simulink model "FinalDemo2021b"  (R2023a)
settings: Solver=VariableStepAuto  StartTime=0.0  StopTime=inf  RelTol=1e-3
settings Model: Creator=bryantboatright  LastModifiedBy=boater

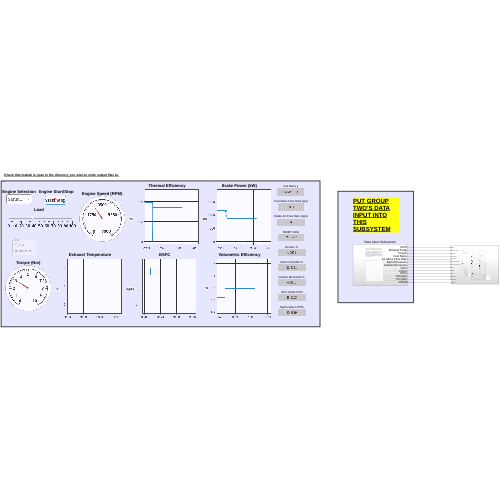
[thumbnail: Simulink's stored preview of the top-level diagram]
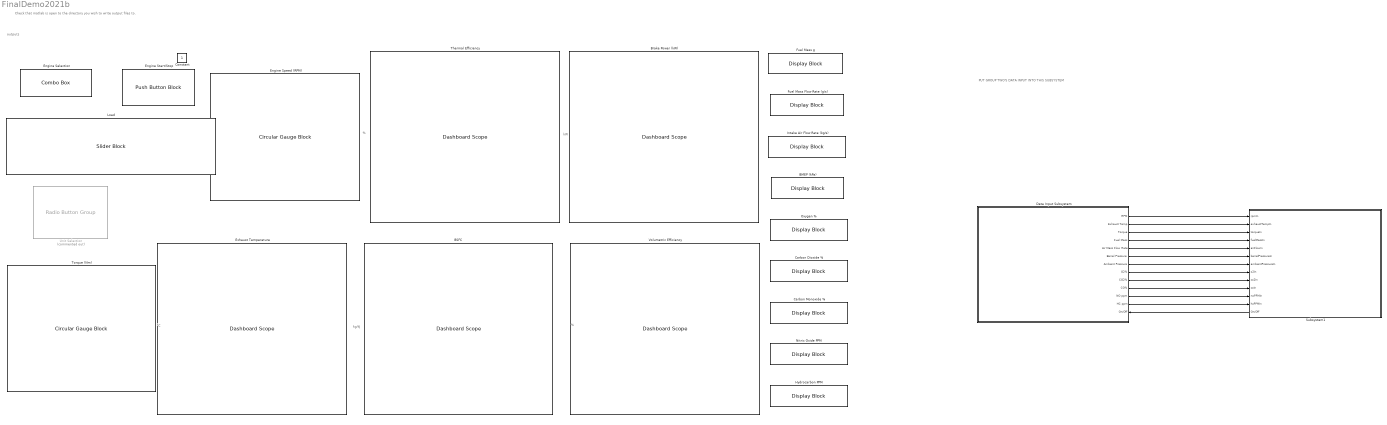
== system FinalDemo2021b ==
  note: %
  note: Check that matlab is open to the directory you wish to write output files to.
  note: PUT GROUP TWO'S DATA INPUT INTO THIS SUBSYSTEM
  note: ˚C
  note: kg/kJ
  note: kW
  note: outputs
  note: %
  BMEP (kPa) : DisplayBlock  LabelPosition=Hide  Transparency=1
  BSFC : DashboardScope  LegendPosition=Hide  UpdateMode=Scroll
  Brake Power (kW) : DashboardScope  LegendPosition=Hide  UpdateMode=Scroll
  Carbon Dioxide % : DisplayBlock  LabelPosition=Hide  Transparency=1
  Carbon Monoxide % : DisplayBlock  LabelPosition=Hide  Transparency=1
  Data Input Subsystem : Subsystem
      settings: PortSchema="{\"entries\":[{\"content\":{\"sides\":[{\"content\":{\"connectorIds\":[]},\"type\":\"ConnectorPlacement.EquallySpacedRectSide\",\"uuid\":\"3754a3e3-4518-42e3-a0cd-0eb816f7e60c\"},{\"content\":{\"connectorIds\":[\"Out1\",\"Out2\",\"Out3\",\"Out4\",\"Out5\",\"Out6\",\"Out7\",\"Out8\",\"Out9\",\"Out10\",\"Out11\",\"Out12\",\"In1\"],\"side\":\"RIGHT\"},\"type\":\"ConnectorPlacement.EquallySpacedRectSide\",\"uuid\":\"d3dfe676-b6e6-4c7f-98c7-8b108f201c07\"},{\"content\":{\"connectorIds\":[],\"side\":\"TOP\"},\"type\":\"ConnectorPlacement.EquallySpacedRectSide\",\"uuid\":\"2f91c8dd-0198-445b-930d-495fc8bcc849\"}]},\"type\":\"ConnectorPlacement.EquallySpacedConnector\",\"uuid\":\"520c6fba-fa44-47d2-96c9-29e04e3d0d93\"}],\"packageUris\":[\"http://schema.mathworks.com/mf0/Connector/R2020b\"],\"version\":\"1.0\"}"
  Engine Selection : ComboBox  LabelPosition=Hide  SelectedLabel=Yanmar
      settings: Values={{'Yanmar', 'Craftsman', 'John Deer', 'Chevy V6', 'Kohler', 'DuroMax'}, [1 2 3 4 5 6]}
  Engine Speed (RPM) : CircularGaugeBlock  LabelPosition=Hide  ScaleMax=7000  TickInterval=1750
  Engine Start/Stop : PushButtonBlock  ButtonText=Start/Stop  ButtonType=Latch  Icon=Engine  IconAlignment=Center  IconColor=On  OffValue=0.000000
  Exhaust Temperature : DashboardScope  LegendPosition=Hide  ScaleAtStop=off
  Fuel Mass Flow Rate (g/s) : DisplayBlock  LabelPosition=Hide  Transparency=1
  Fuel Mass g : DisplayBlock  LabelPosition=Hide  Transparency=1
  Hydrocarbon PPM : DisplayBlock  LabelPosition=Hide  Transparency=1
  Intake Air Flow Rate (kg/s) : DisplayBlock  LabelPosition=Hide  Transparency=1
  Load : SliderBlock  LabelPosition=Hide
  Nitric Oxide PPM : DisplayBlock  LabelPosition=Hide  Transparency=1
  Oxygen % : DisplayBlock  LabelPosition=Hide  Transparency=1
  Subsystem1 : Subsystem
      settings: PortSchema="{\"entries\":[{\"content\":{\"sides\":[{\"content\":{\"connectorIds\":[\"In1\",\"In2\",\"In3\",\"In4\",\"In5\",\"In6\",\"In7\",\"In8\",\"In9\",\"In10\",\"In11\",\"In12\",\"Out1\"]},\"type\":\"ConnectorPlacement.EquallySpacedRectSide\",\"uuid\":\"2e8fbbbd-04f3-4cfb-b1cc-1db1e48dc879\"},{\"content\":{\"connectorIds\":[],\"side\":\"RIGHT\"},\"type\":\"ConnectorPlacement.EquallySpacedRectSide\",\"uuid\":\"1e86395c-1e99-406b-884b-92366c924b1f\"},{\"content\":{\"connectorIds\":[],\"side\":\"TOP\"},\"type\":\"ConnectorPlacement.EquallySpacedRectSide\",\"uuid\":\"23f1f2f5-9354-4dfe-ba19-9e9e16993f9b\"}]},\"type\":\"ConnectorPlacement.EquallySpacedConnector\",\"uuid\":\"bb08251b-5f96-4a99-a638-0e0833315a09\"}],\"packageUris\":[\"http://schema.mathworks.com/mf0/Connector/R2020b\"],\"version\":\"1.0\"}"
  Thermal Efficiency : DashboardScope  LegendPosition=Hide  UpdateMode=Scroll
  Torque (Nm) : CircularGaugeBlock  LabelPosition=Hide  ScaleMax=10  TickInterval=1
  Unit Selection : RadioButtonGroup  Commented=on  LabelPosition=Hide  SelectedLabel=Imperial  ButtonGroupName=Units
      settings: Values={{'Metric', 'Imperial'}, [0 1]}
  Volumetric Efficiency : DashboardScope  LegendPosition=Hide  UpdateMode=Scroll
  Constant : Constant  IOType=siggen
  wires:
  Data Input Subsystem/1(RPM) -> Subsystem1/1(rpmIn)
  Data Input Subsystem/2(Exhaust Temp) -> Subsystem1/2(exhaustTempIn)
  Data Input Subsystem/3(Torque) -> Subsystem1/3(torqueIn)
  Data Input Subsystem/4(Fuel Mass) -> Subsystem1/4(fuelMassIn)
  Data Input Subsystem/5(Air Mass Flow Rate) -> Subsystem1/5(airFlowIn)
  Data Input Subsystem/6(Barrel Pressure) -> Subsystem1/6(barrelPressureIn)
  Data Input Subsystem/7(Ambient Pressure) -> Subsystem1/7(ambientPressureIn)
  Data Input Subsystem/8(O2%) -> Subsystem1/8(o2In)
  Data Input Subsystem/9(CO2%) -> Subsystem1/9(co2In)
  Data Input Subsystem/10(CO%) -> Subsystem1/10(coIn)
  Data Input Subsystem/11(NO ppm) -> Subsystem1/11(noPPMIn)
  Data Input Subsystem/12(HC ppm) -> Subsystem1/12(hcPPMIn)
  Subsystem1/1(On/Off) -> Data Input Subsystem/1(On/Off)

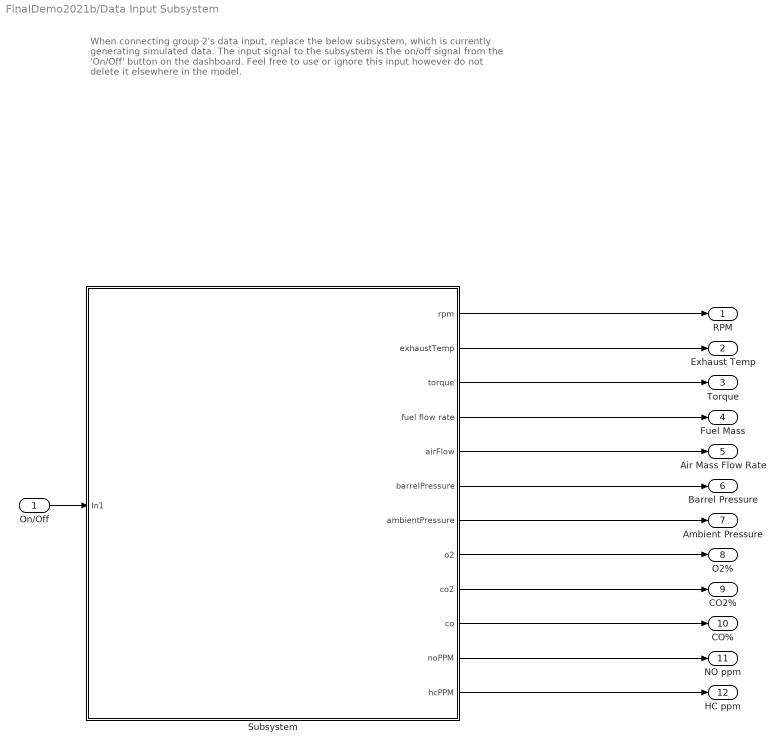
== system FinalDemo2021b/Data Input Subsystem ==
  note: When connecting group 2's data input, replace the below subsystem, which is currently generating simulated data. The input signal to the subsystem is the on/off signal from the 'On/Off' button on the dashboard. Feel free to use or ignore this input however do not delete it elsewhere in the model.
  On/Off : Inport
  Subsystem : Subsystem
  RPM : Outport
  Exhaust Temp : Outport  Port=2
  Torque : Outport  Port=3
  Fuel Mass : Outport  Port=4
  Air Mass Flow Rate : Outport  Port=5
  Barrel Pressure : Outport  Port=6
  Ambient Pressure : Outport  Port=7
  O2% : Outport  Port=8
  CO2% : Outport  Port=9
  CO% : Outport  Port=10
  NO ppm : Outport  Port=11
  HC ppm : Outport  Port=12
  wires:
  Subsystem/1(rpm) -> RPM/1
  Subsystem/2(exhaustTemp) -> Exhaust Temp/1
  Subsystem/3(torque) -> Torque/1
  Subsystem/4(fuel flow rate) -> Fuel Mass/1
  Subsystem/5(airFlow) -> Air Mass Flow Rate/1
  Subsystem/6(barrelPressure) -> Barrel Pressure/1
  Subsystem/7(ambientPressure) -> Ambient Pressure/1
  Subsystem/8(o2) -> O2%/1
  Subsystem/9(co2) -> CO2%/1
  Subsystem/10(co) -> CO%/1
  Subsystem/11(noPPM) -> NO ppm/1
  Subsystem/12(hcPPM) -> HC ppm/1
  On/Off/1 -> Subsystem/1(In1)

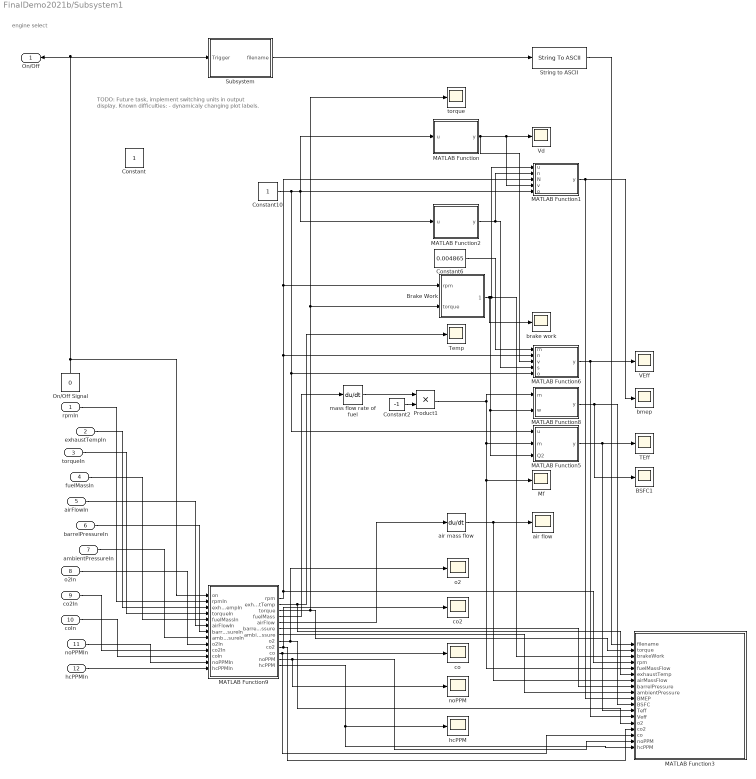
== system FinalDemo2021b/Subsystem1 ==
  note: TODO: Future task, implement switching units in output display.
      |
      | Known difficulties:
      | - dynamicaly changing plot labels.
  note: engine select
  rpmIn : Inport
  exhaustTempIn : Inport  Port=2
  torqueIn : Inport  Port=3
  fuelMassIn : Inport  Port=4
  airFlowIn : Inport  Port=5
  barrelPressureIn : Inport  Port=6
  ambientPressureIn : Inport  Port=7
  o2In : Inport  Port=8
  co2In : Inport  Port=9
  coIn : Inport  Port=10
  noPPMIn : Inport  Port=11
  hcPPMIn : Inport  Port=12
  BSFC1 : Scope
  Brake Work : MATLAB Function  TreatAsAtomicUnit=on
  Constant : Constant
  Constant10 : Constant
  Constant2 : Constant  Value=-1
  Constant6 : Constant  Value=0.004865
  MATLAB Function : MATLAB Function  TreatAsAtomicUnit=on
  MATLAB Function1 : MATLAB Function  TreatAsAtomicUnit=on
  MATLAB Function2 : MATLAB Function  TreatAsAtomicUnit=on
  MATLAB Function3 : MATLAB Function  TreatAsAtomicUnit=on
  MATLAB Function5 : MATLAB Function  TreatAsAtomicUnit=on
  MATLAB Function6 : MATLAB Function  TreatAsAtomicUnit=on
  MATLAB Function8 : MATLAB Function  TreatAsAtomicUnit=on
  MATLAB Function9 : MATLAB Function  TreatAsAtomicUnit=on
  Mf : Scope
  On/Off Signal : Constant  Value=0
  Product1 : Product
  String to ASCII : StringToASCII
  Subsystem : Subsystem
  TEff : Scope
  Temp : Scope
  VEff : Scope
  Vd : Scope
  air flow : Scope
  air mass flow : Derivative
  bmep : Scope
  brake work : Scope
  co : Scope
  co2 : Scope
  hcPPM : Scope
  mass flow rate of fuel : Derivative
  noPPM : Scope
  o2 : Scope
  torque : Scope
  On/Off : Outport
  wires:
  MATLAB Function5/1(y) -> TEff/1, MATLAB Function3/12(Teff)
  MATLAB Function6/1(y) -> VEff/1, MATLAB Function3/13(Veff)
  air mass flow/1 -> air flow/1, MATLAB Function3/7(airMassFlow)
  Brake Work/1(brakeWork) -> MATLAB Function8/2(w), MATLAB Function5/3(Q2), MATLAB Function1/1(u), MATLAB Function3/3(brakeWork), brake work/1
  MATLAB Function8/1(y) -> BSFC1/1, MATLAB Function3/11(BSFC)
  MATLAB Function2/1(y) -> MATLAB Function1/2(n), MATLAB Function6/4(s)
  Constant6/1 -> MATLAB Function6/1(m)
  MATLAB Function/1(y) -> MATLAB Function1/4(v), Vd/1, MATLAB Function6/3(v)
  MATLAB Function9/12(hcPPM) -> hcPPM/1, MATLAB Function3/18(hcPPM)
  MATLAB Function9/11(noPPM) -> noPPM/1, MATLAB Function3/17(noPPM)
  MATLAB Function9/10(co) -> co/1, MATLAB Function3/16(co)
  MATLAB Function9/9(co2) -> co2/1, MATLAB Function3/15(co2)
  hcPPMIn/1 -> MATLAB Function9/13(hcPPMIn)
  MATLAB Function9/4(fuelMass) -> mass flow rate of fuel/1
  MATLAB Function9/1(rpm) -> Brake Work/1(rpm), MATLAB Function1/3(N), MATLAB Function6/2(n), MATLAB Function3/4(rpm)
  Subsystem/1(filename) -> String to ASCII/1
  MATLAB Function9/8(o2) -> o2/1, MATLAB Function3/14(o2)
  MATLAB Function1/1(y) -> bmep/1, MATLAB Function3/10(BMEP)
  noPPMIn/1 -> MATLAB Function9/12(noPPMIn)
  MATLAB Function9/3(torque) -> torque/1, Brake Work/2(torque), MATLAB Function3/2(torque)
  coIn/1 -> MATLAB Function9/11(coIn)
  Constant10/1 -> MATLAB Function5/1(u), MATLAB Function6/5(o), MATLAB Function/1(u), MATLAB Function2/1(u), MATLAB Function1/5(o)
  MATLAB Function9/2(exhaustTemp) -> Temp/1, MATLAB Function3/6(exhaustTemp)
  co2In/1 -> MATLAB Function9/10(co2In)
  exhaustTempIn/1 -> MATLAB Function9/3(exhaustTempIn)
  ambientPressureIn/1 -> MATLAB Function9/8(ambientPressureIn)
  MATLAB Function9/6(barrelPressure) -> MATLAB Function3/8(barrelPressure)
  rpmIn/1 -> MATLAB Function9/2(rpmIn)
  MATLAB Function9/7(ambientPressure) -> MATLAB Function3/9(ambientPressure)
  fuelMassIn/1 -> MATLAB Function9/5(fuelMassIn)
  String to ASCII/1 -> MATLAB Function3/1(filename)
  MATLAB Function9/5(airFlow) -> air mass flow/1
  o2In/1 -> MATLAB Function9/9(o2In)
  barrelPressureIn/1 -> MATLAB Function9/7(barrelPressureIn)
  torqueIn/1 -> MATLAB Function9/4(torqueIn)
  airFlowIn/1 -> MATLAB Function9/6(airFlowIn)
  On/Off Signal/1 -> Subsystem/1(Trigger), On/Off/1, MATLAB Function9/1(on)
  Constant2/1 -> Product1/2
  Product1/1 -> MATLAB Function8/1(m), MATLAB Function3/5(fuelMassFlow), Mf/1, MATLAB Function5/2(m)
  mass flow rate of fuel/1 -> Product1/1

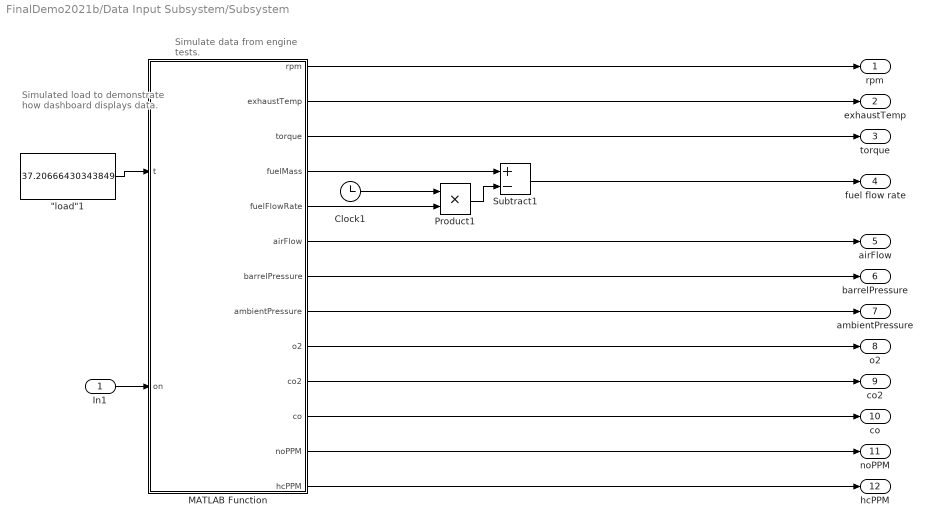
== system FinalDemo2021b/Data Input Subsystem/Subsystem ==
  note: Simulated load to demonstrate how
      | dashboard displays data.
  note: Simulate data from engine
      | tests.
  In1 : Inport
  "\"load\"1" : Constant  Value=37.20666430343849
  Clock1 : Clock
  MATLAB Function : MATLAB Function  TreatAsAtomicUnit=on
  Product1 : Product
  Subtract1 : Sum  Inputs=+-
  rpm : Outport
  exhaustTemp : Outport  Port=2
  torque : Outport  Port=3
  fuel flow rate : Outport  Port=4
  airFlow : Outport  Port=5
  barrelPressure : Outport  Port=6
  ambientPressure : Outport  Port=7
  o2 : Outport  Port=8
  co2 : Outport  Port=9
  co : Outport  Port=10
  noPPM : Outport  Port=11
  hcPPM : Outport  Port=12
  wires:
  MATLAB Function/3(torque) -> torque/1
  MATLAB Function/13(hcPPM) -> hcPPM/1
  MATLAB Function/1(rpm) -> rpm/1
  MATLAB Function/6(airFlow) -> airFlow/1
  MATLAB Function/5(fuelFlowRate) -> Product1/2
  MATLAB Function/12(noPPM) -> noPPM/1
  MATLAB Function/7(barrelPressure) -> barrelPressure/1
  MATLAB Function/8(ambientPressure) -> ambientPressure/1
  In1/1 -> MATLAB Function/2(on)
  MATLAB Function/9(o2) -> o2/1
  MATLAB Function/2(exhaustTemp) -> exhaustTemp/1
  "\"load\"1"/1 -> MATLAB Function/1(t)
  MATLAB Function/4(fuelMass) -> Subtract1/1
  MATLAB Function/11(co) -> co/1
  MATLAB Function/10(co2) -> co2/1
  Product1/1 -> Subtract1/2
  Clock1/1 -> Product1/1
  Subtract1/1 -> fuel flow rate/1

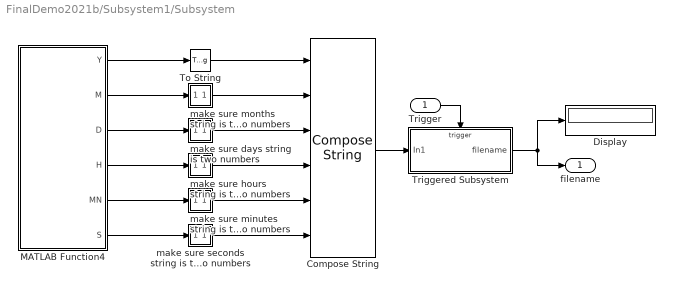
== system FinalDemo2021b/Subsystem1/Subsystem ==
  Trigger : Inport
  Compose String : ComposeString  Format="\"%s-%s-%s--%s-%s-%s-output.csv\""
  Display : Display
  MATLAB Function4 : MATLAB Function  TreatAsAtomicUnit=on  SystemSampleTime=200
  To String : ToString
  Triggered Subsystem : Subsystem  TreatAsAtomicUnit=on
  make sure days string is two numbers : Subsystem
  make sure hours string is two numbers : Subsystem
  make sure minutes string is two numbers : Subsystem
  make sure months string is two numbers : Subsystem
  make sure seconds string is two numbers : Subsystem
  filename : Outport
  wires:
  make sure months string is two numbers/1(Out1) -> Compose String/2
  To String/1 -> Compose String/1
  MATLAB Function4/6(S) -> make sure seconds string is two numbers/1(In1)
  Compose String/1 -> Triggered Subsystem/1(In1)
  MATLAB Function4/5(MN) -> make sure minutes string is two numbers/1(In1)
  make sure days string is two numbers/1(Out1) -> Compose String/3
  make sure minutes string is two numbers/1(Out1) -> Compose String/5
  MATLAB Function4/4(H) -> make sure hours string is two numbers/1(In1)
  make sure hours string is two numbers/1(Out1) -> Compose String/4
  Trigger/1 -> Triggered Subsystem/Trigger
  MATLAB Function4/2(M) -> make sure months string is two numbers/1(In1)
  Triggered Subsystem/1(filename) -> filename/1, Display/1
  MATLAB Function4/3(D) -> make sure days string is two numbers/1(In1)
  MATLAB Function4/1(Y) -> To String/1
  make sure seconds string is two numbers/1(Out1) -> Compose String/6

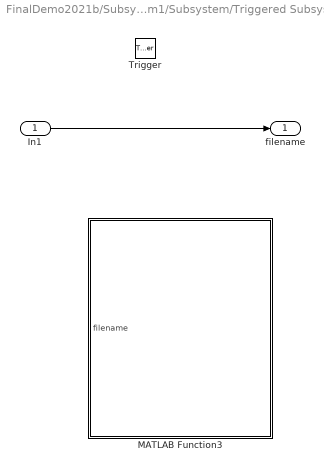
== system FinalDemo2021b/Subsystem1/Subsystem/Triggered Subsystem ==
  In1 : Inport
  Trigger : TriggerPort  VariantControl=(inherit)
  MATLAB Function3 : MATLAB Function  TreatAsAtomicUnit=on
  filename : Outport
  wires:
  In1/1 -> filename/1

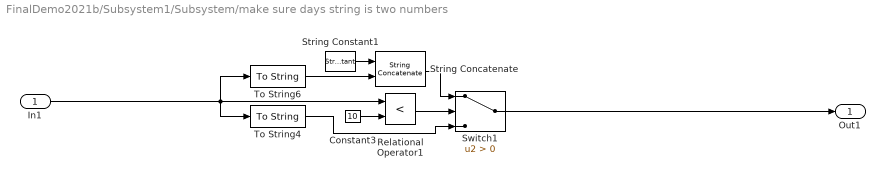
== system FinalDemo2021b/Subsystem1/Subsystem/make sure days string is two numbers ==
  In1 : Inport
  Constant3 : Constant  Value=10  VectorParams1D=off  OutDataTypeStr=int8
  Relational Operator1 : RelationalOperator  Operator=<  OutDataTypeStr=boolean  RndMeth=Simplest  InputSameDT=off
  String Concatenate : StringConcatenate
  String Constant1 : StringConstant  String="\"0\""
  Switch1 : Switch  Criteria=u2 > Threshold  SaturateOnIntegerOverflow=off  InputSameDT=off
  To String4 : ToString
  To String6 : ToString
  Out1 : Outport
  wires:
  Constant3/1 -> Relational Operator1/2
  Relational Operator1/1 -> Switch1/2
  To String4/1 -> Switch1/3
  To String6/1 -> String Concatenate/2
  String Constant1/1 -> String Concatenate/1
  String Concatenate/1 -> Switch1/1
  In1/1 -> Relational Operator1/1, To String4/1, To String6/1
  Switch1/1 -> Out1/1

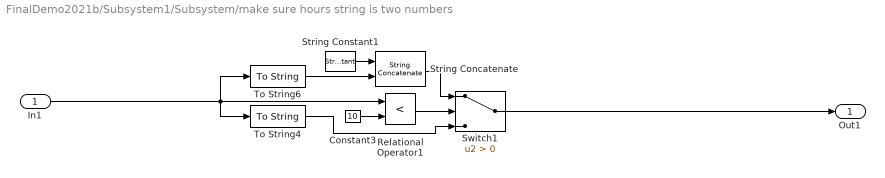
== system FinalDemo2021b/Subsystem1/Subsystem/make sure hours string is two numbers ==
  In1 : Inport
  Constant3 : Constant  Value=10  VectorParams1D=off  OutDataTypeStr=int8
  Relational Operator1 : RelationalOperator  Operator=<  OutDataTypeStr=boolean  RndMeth=Simplest  InputSameDT=off
  String Concatenate : StringConcatenate
  String Constant1 : StringConstant  String="\"0\""
  Switch1 : Switch  Criteria=u2 > Threshold  SaturateOnIntegerOverflow=off  InputSameDT=off
  To String4 : ToString
  To String6 : ToString
  Out1 : Outport
  wires:
  Switch1/1 -> Out1/1
  In1/1 -> To String6/1, To String4/1, Relational Operator1/1
  String Concatenate/1 -> Switch1/1
  String Constant1/1 -> String Concatenate/1
  To String6/1 -> String Concatenate/2
  To String4/1 -> Switch1/3
  Relational Operator1/1 -> Switch1/2
  Constant3/1 -> Relational Operator1/2

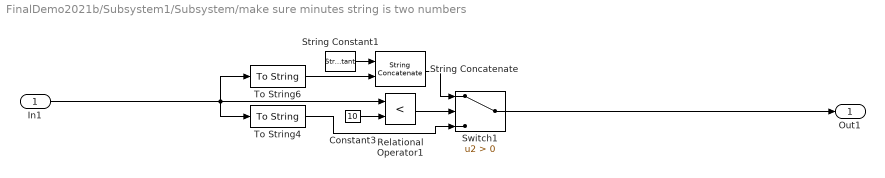
== system FinalDemo2021b/Subsystem1/Subsystem/make sure minutes string is two numbers ==
  In1 : Inport
  Constant3 : Constant  Value=10  VectorParams1D=off  OutDataTypeStr=int8
  Relational Operator1 : RelationalOperator  Operator=<  OutDataTypeStr=boolean  RndMeth=Simplest  InputSameDT=off
  String Concatenate : StringConcatenate
  String Constant1 : StringConstant  String="\"0\""
  Switch1 : Switch  Criteria=u2 > Threshold  SaturateOnIntegerOverflow=off  InputSameDT=off
  To String4 : ToString
  To String6 : ToString
  Out1 : Outport
  wires:
  Constant3/1 -> Relational Operator1/2
  Relational Operator1/1 -> Switch1/2
  To String4/1 -> Switch1/3
  To String6/1 -> String Concatenate/2
  String Constant1/1 -> String Concatenate/1
  String Concatenate/1 -> Switch1/1
  In1/1 -> Relational Operator1/1, To String4/1, To String6/1
  Switch1/1 -> Out1/1

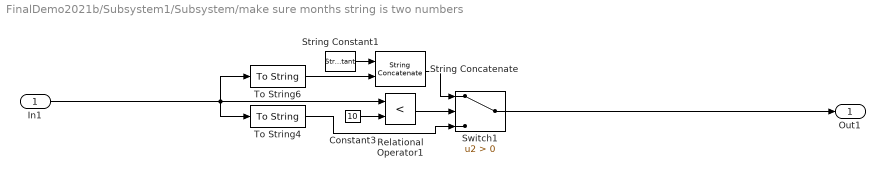
== system FinalDemo2021b/Subsystem1/Subsystem/make sure months string is two numbers ==
  In1 : Inport
  Constant3 : Constant  Value=10  VectorParams1D=off  OutDataTypeStr=int8
  Relational Operator1 : RelationalOperator  Operator=<  OutDataTypeStr=boolean  RndMeth=Simplest  InputSameDT=off
  String Concatenate : StringConcatenate
  String Constant1 : StringConstant  String="\"0\""
  Switch1 : Switch  Criteria=u2 > Threshold  SaturateOnIntegerOverflow=off  InputSameDT=off
  To String4 : ToString
  To String6 : ToString
  Out1 : Outport
  wires:
  Switch1/1 -> Out1/1
  In1/1 -> To String6/1, To String4/1, Relational Operator1/1
  String Concatenate/1 -> Switch1/1
  String Constant1/1 -> String Concatenate/1
  To String6/1 -> String Concatenate/2
  To String4/1 -> Switch1/3
  Relational Operator1/1 -> Switch1/2
  Constant3/1 -> Relational Operator1/2

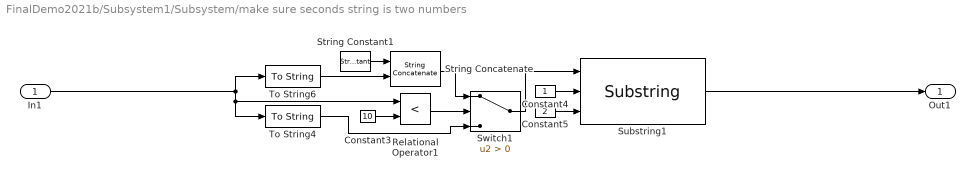
== system FinalDemo2021b/Subsystem1/Subsystem/make sure seconds string is two numbers ==
  In1 : Inport
  Constant3 : Constant  Value=10  VectorParams1D=off  OutDataTypeStr=int8
  Constant4 : Constant  VectorParams1D=off  OutDataTypeStr=int8
  Constant5 : Constant  Value=2  VectorParams1D=off  OutDataTypeStr=uint8
  Relational Operator1 : RelationalOperator  Operator=<  OutDataTypeStr=boolean  RndMeth=Simplest  InputSameDT=off
  String Concatenate : StringConcatenate
  String Constant1 : StringConstant  String="\"0\""
  Substring1 : Substring
  Switch1 : Switch  Criteria=u2 > Threshold  SaturateOnIntegerOverflow=off  InputSameDT=off
  To String4 : ToString
  To String6 : ToString
  Out1 : Outport
  wires:
  Substring1/1 -> Out1/1
  To String4/1 -> Switch1/3
  Switch1/1 -> Substring1/1
  Constant3/1 -> Relational Operator1/2
  Constant5/1 -> Substring1/3
  In1/1 -> Relational Operator1/1, To String4/1, To String6/1
  Constant4/1 -> Substring1/2
  Relational Operator1/1 -> Switch1/2
  To String6/1 -> String Concatenate/2
  String Constant1/1 -> String Concatenate/1
  String Concatenate/1 -> Switch1/1

== matlab function FinalDemo2021b/Subsystem1/MATLAB Function6 ==
  data: m input; y output; n input; v input; s input; o input
function y = fcn(m, n, v, s,o)
if(o == 1 || o == 2 || o == 5 || o == 6)
    y = ((s*m)/(1.205*v*(n/60)));
elseif (o == 3)
    y = ((s*m)/(1.205*(v*4)*(n/60)));
else
    y = ((s*m)/(1.205*(v*6)*(n/60)));
end

== matlab function FinalDemo2021b/Subsystem1/Subsystem/MATLAB Function4 ==
  data: Y output; M output; D output; H output; MN output; S output
function [Y, M, D, H, MN, S] = dateGenerator()
   coder.extrinsic('now');
   coder.extrinsic('datevec');
   Y = 0;
   M = 0;
   D = 0;
   H = 0;
   MN = 0;
   S = 0;
   [Y, M, D, H, MN, S] = datevec(datetime("now"));
end

== matlab function FinalDemo2021b/Subsystem1/MATLAB Function8 ==
  data: m input; y output; w input
function y = fcn(m,w)

y = m./w;

== matlab function FinalDemo2021b/Subsystem1/MATLAB Function9 ==
  data: rpm output; exhaustTemp output; torque output; fuelMass output; airFlow output; barrelPressure output; ambientPressure output; on input; o2 output; co2 output; co output; noPPM output; hcPPM output; rpmIn input; exhaustTempIn input; torqueIn input; fuelMassIn input; airFlowIn input; barrelPressureIn input; ambientPressureIn input; o2In input; co2In input; coIn input; noPPMIn input; hcPPMIn input
% function to take input of 
%
% returns:
%
%   rpm: engine     speed rev per minute
%   exhaustTemp:    exhaust temperature in celsius
%   torque:         torque in Newton-meters
%   torqueMeasured: boolean - true if torque is measured, false if not
%   volts:          voltage
%   amps:           current
%   fuelMass:       mass of fuel container at current time.
%   

function [ rpm,exhaustTemp,torque,fuelMass,airFlow,barrelPressure,ambientPressure,...
    o2,co2,co,noPPM,hcPPM ] = fcn(on,rpmIn,exhaustTempIn,torqueIn,fuelMassIn,...
    airFlowIn,barrelPressureIn,ambientPressureIn,o2In,co2In,coIn,noPPMIn,hcPPMIn)
if(on == 1)
    rpm = rpmIn;
    exhaustTemp = exhaustTempIn;
    torque = torqueIn;
    fuelMass = fuelMassIn;
    airFlow = airFlowIn;
    barrelPressure = barrelPressureIn;
    ambientPressure = ambientPressureIn;
    o2 = o2In;
    co2 = co2In;
    co = coIn;
    noPPM = noPPMIn;
    hcPPM = hcPPMIn;
else
    rpm = 0;
    exhaustTemp = 0;
    torque = 0;
    fuelMass = 0;
    airFlow = 0;
    barrelPressure = 0;
    ambientPressure = 0;
    o2 = 0;
    co2 = 0;
    co = 0;
    noPPM = 0;
    hcPPM = 0;
end

== matlab function FinalDemo2021b/Subsystem1/MATLAB Function3 ==
  data: filename input; torque input; brakeWork input; rpm input; fuelMassFlow input; exhaustTemp input; airMassFlow input; barrelPressure input; ambientPressure input; BMEP input; BSFC input; Teff input; Veff input; o2 input; co2 input; co input; noPPM input; hcPPM input
% log file generation - currently overwrites each run
% \r\n used for windows line termination style CRLF - switch to just \n if
% using unix like system
function fileOutput(filename,torque,brakeWork,rpm,fuelMassFlow,exhaustTemp,airMassFlow,barrelPressure,ambientPressure,BMEP,BSFC,Teff,Veff,o2,co2,co,noPPM,hcPPM)

if ([0 0] ~= size(double(char(filename))))
    file = fopen(char(filename),'a');
    if (0 > file)
        return
    end

    fprintf(file,'%.3f,%.3f,%.3f,%.3f,%.3f,%.3f,%.3f,%.3f,%.3f,%.3f,%.3f,%.3f,%.3f,%.3f,%.3f,%.3f,%.3f\r\n', ...
        torque,brakeWork,rpm,fuelMassFlow,exhaustTemp,airMassFlow,barrelPressure,ambientPressure,BMEP,BSFC,Teff,Veff,o2,co2,co,noPPM,hcPPM);
    fclose(file);
end

== matlab function FinalDemo2021b/Subsystem1/Subsystem/Triggered Subsystem/MATLAB Function3 ==
  data: filename input
% log file generation - currently overwrites each run
% \r\n used for windows line termination style CRLF - switch to just \n if
% using unix like system
function fileOutput(filename)

if ([0 0] ~= size(double(char(filename))))
    file = fopen(char(filename),'a');
    if (0 > file)
        return
    end

    fprintf(file,['torque,brakeWork,rpm,fuel mass flow,exhaust temperature,air mass flow..' ...
        ',barrel pressure,ambient pressure,BMEP,BSFC,thermal efficiency,...' ...
        'volumetric efficiency,o2,co2,co,no PPM,hc PPM\r\n']);
    fclose(file);
end

== matlab function FinalDemo2021b/Subsystem1/MATLAB Function1 ==
  data: u input; y output; n input; N input; v input; o input
function y = fcn(u, n, N,  v, o)
if(o == 1 || o == 2 || o == 5 || o ==6)
    y = ((u/((N/60)/n))/v)/1000;
elseif(o==3)
     y = ((u/((N/60)/n))/(v*4))/1000;
else
     y = ((u/((N/60)/n))/(v*6))/1000;
end

== matlab function FinalDemo2021b/Subsystem1/MATLAB Function ==
  data: y output; u input
function y = fcn(u)
data = [0.000296 0.000196 0.000475 000.0004667 0.000429 0.000225];

y = data(1,u);

== matlab function FinalDemo2021b/Subsystem1/MATLAB Function2 ==
  data: y output; u input
function y = fcn(u)
data = [4  4  4  4 4 4];

y = data(1,u);

== matlab function FinalDemo2021b/Subsystem1/Brake Work ==
  data: rpm input; brakeWork output; torque input
function brakeWork = fcn(rpm,torque)
brakeWork = 2 * pi * (rpm/60.0) * torque;

== matlab function FinalDemo2021b/Data Input Subsystem/Subsystem/MATLAB Function ==
  data: t input; rpm output; on input; exhaustTemp output; torque output; fuelMass output; fuelFlowRate output; airFlow output; barrelPressure output; ambientPressure output; o2 output; co2 output; co output; noPPM output; hcPPM output
function [ rpm,exhaustTemp,torque,fuelMass,fuelFlowRate,airFlow,barrelPressure,ambientPressure,...
    o2,co2,co,noPPM,hcPPM ] = fcn(t,on)
if (on)
    data = (1 + t / 100.0) * [ 2000 125 2.258 2000.0 0.004 0.94 3.4 16.5 0.003 35 59 0.004 ];
    rpm = data(1);
    exhaustTemp = data(2);
    torque = data(3);
    fuelMass = data(4);
    airFlow = data(5);
    barrelPressure = data(6);
    ambientPressure = 29;
    o2 = data(7);
    co2 = data(8);
    co = data(9);
    noPPM = data(10);
    hcPPM = data(11);
    fuelFlowRate = data(12);
else
    rpm = 0;
    exhaustTemp = 0;
    torque = 0;
    fuelMass = 0;
    airFlow = 0;
    barrelPressure = 0;
    ambientPressure = 0;
    o2 = 0;
    co2 = 0;
    co = 0;
    noPPM = 0;
    hcPPM = 0;
    fuelFlowRate = 0;
end

== matlab function FinalDemo2021b/Subsystem1/MATLAB Function5 ==
  data: y output; u input; m input; Q2 input
function y = fcn(u, m, Q2)
data = [47.3e6 44.4e6];
Q1 = 0;
if(u == 3)
    Q1 = m * data(1, 2);

else
    Q1 = m * data(1,1);
end

y = (Q2/Q1) * 100;
